simulink model "DC Motor Transfer Function Model"  (R2023b)
settings: Solver=VariableStepAuto  StartTime=0.0  StopTime=20.0  RelTol=1e-3
InitFcn:
  | Jm=0.000052;
  | Bm=0.01;
  | Kb=0.235;
  | Kt=0.235;
  | Ra=2;
  | La=0.23

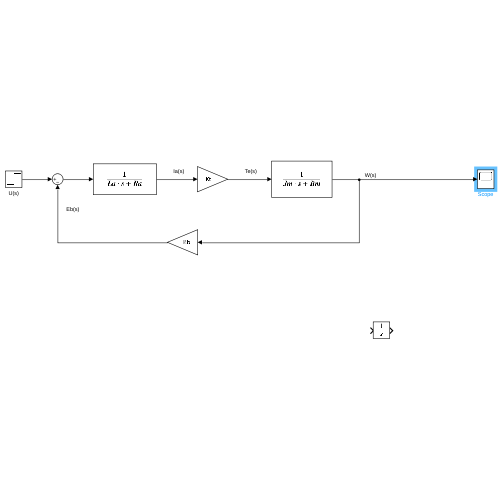
[thumbnail: Simulink's stored preview of the top-level diagram]
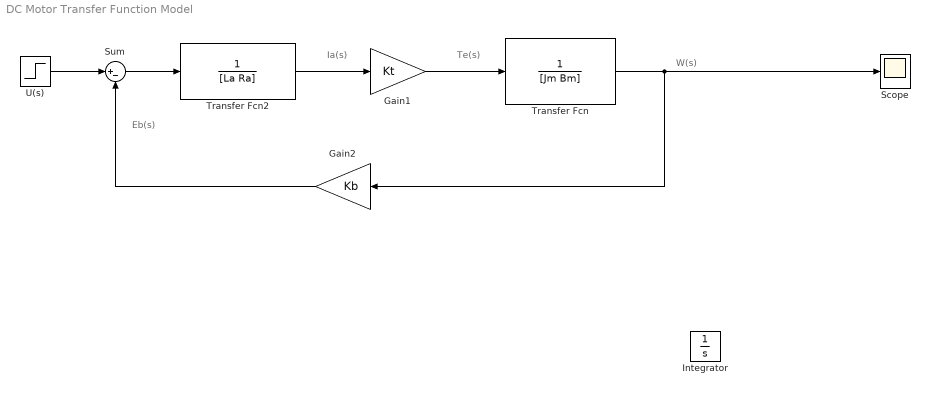
== system DC Motor Transfer Function Model ==
  note: Eb(s)
  note: W(s)
  note: Te(s)
  note: Ia(s)
  Gain1 : Gain  Gain=Kt
  Gain2 : Gain  Gain=Kb
  Integrator : Integrator
  Scope : Scope
  Sum : Sum  Inputs=|+-
  Transfer Fcn : TransferFcn  Denominator=[Jm Bm]
  Transfer Fcn2 : TransferFcn  Denominator=[La Ra]
  U(s) : Step  Time=2  After=5  SampleTime=0
  wires:
  Sum/1 -> Transfer Fcn2/1
  Transfer Fcn2/1 -> Gain1/1
  Gain1/1 -> Transfer Fcn/1
  Transfer Fcn/1 -> Gain2/1, Scope/1
  Gain2/1 -> Sum/2
  U(s)/1 -> Sum/1
